simulink model "Phase1_Controller"  (R2024b)
settings: Solver=VariableStepAuto  StartTime=0.0  StopTime=10.0  RelTol=1e-3
values from neighbouring files (symbols this model uses):
  I_link = 0.15    [variables.mat]
  K_limit = 50    [variables.mat]
  L_com = 0.3    [variables.mat]
  m_link = 2    [variables.mat]
  thetha_max_soft = 85    [variables.mat]
  thetha_min_soft = 5    [variables.mat]
settings Model: Creator=ranica  LastModifiedBy=rorysucharov-gluck

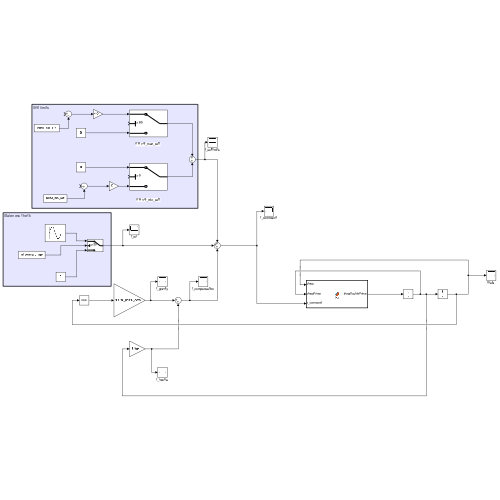
[thumbnail: Simulink's stored preview of the top-level diagram]
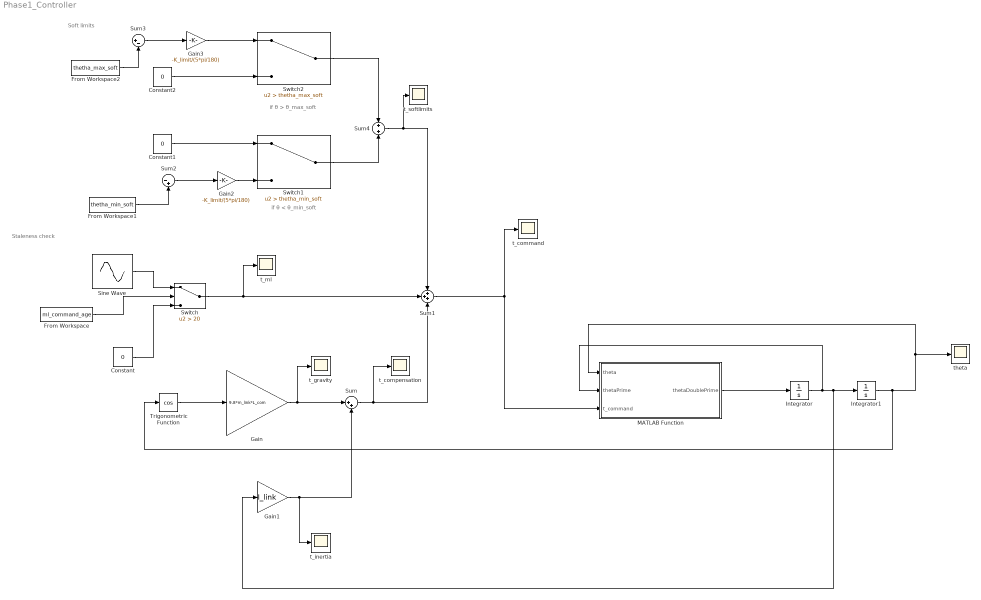
== system Phase1_Controller ==
  note: Soft limits
  note: Staleness check
  note: if θ > θ_max_soft
  note: if θ < θ_min_soft
  Constant : Constant  Value=0
  Constant1 : Constant  Value=0
  Constant2 : Constant  Value=0
  From Workspace : FromWorkspace  VariableName=ml_command_age
  From Workspace1 : FromWorkspace  VariableName=thetha_min_soft
  From Workspace2 : FromWorkspace  VariableName=thetha_max_soft
  Gain : Gain  Gain=9.8*m_link*L_com
  Gain1 : Gain  Gain=I_link
  Gain2 : Gain  Gain=-K_limit/(5*pi/180)
  Gain3 : Gain  Gain=-K_limit/(5*pi/180)
  Integrator : Integrator
  Integrator1 : Integrator
  MATLAB Function : MATLAB Function  TreatAsAtomicUnit=on
  Sine Wave : Sin  Frequency=2*pi*100  SampleTime=0
  Sum : Sum  Inputs=|++
  Sum1 : Sum  Inputs=+++
  Sum2 : Sum  Inputs=|-+
  Sum3 : Sum  Inputs=|+-
  Sum4 : Sum  Inputs=+|+
  Switch : Switch  Criteria=u2 > Threshold  Threshold=20  SaturateOnIntegerOverflow=off  InputSameDT=off
  Switch1 : Switch  Criteria=u2 > Threshold  Threshold=thetha_min_soft  SaturateOnIntegerOverflow=off  InputSameDT=off
  Switch2 : Switch  Criteria=u2 > Threshold  Threshold=thetha_max_soft  SaturateOnIntegerOverflow=off  InputSameDT=off
  Trigonometric Function : Trigonometry  Operator=cos
  t_command : Scope
  t_compensation : Scope
  t_gravity : Scope
  t_inertia : Scope
  t_ml : Scope
  t_softlimits : Scope
  theta : Scope
  wires:
  Sine Wave/1 -> Switch/1
  Constant/1 -> Switch/3
  From Workspace/1 -> Switch/2
  Trigonometric Function/1 -> Gain/1
  Gain/1 -> t_gravity/1, Sum/1
  Gain1/1 -> Sum/2, t_inertia/1
  Sum/1 -> Sum1/3, t_compensation/1
  Switch/1 -> t_ml/1, Sum1/2
  Constant1/1 -> Switch1/1
  From Workspace1/1 -> Sum2/2
  Gain2/1 -> Switch1/3
  Sum2/1 -> Gain2/1
  Constant2/1 -> Switch2/3
  Gain3/1 -> Switch2/1
  From Workspace2/1 -> Sum3/2
  Sum3/1 -> Gain3/1
  Switch2/1 -> Sum4/1
  Sum4/1 -> t_softlimits/1, Sum1/1
  Switch1/1 -> Sum4/2
  Sum1/1 -> MATLAB Function/3(t_command), t_command/1
  Integrator1/1 -> theta/1, MATLAB Function/1(theta), Trigonometric Function/1
  MATLAB Function/1(thetaDoublePrime) -> Integrator/1
  Integrator/1 -> MATLAB Function/2(thetaPrime), Gain1/1, Integrator1/1

== matlab function Phase1_Controller/MATLAB Function ==
  data: theta input; thetaDoublePrime output; thetaPrime input; t_command input
function thetaDoublePrime = fnc(theta, thetaPrime, t_command)

thetaDoublePrime = ((t_command - t_gravity_load - D_friction*thetaPrime)) / (I_link + I_joint);
